simulink model "Training_Model_compactHEMS"  (R2023b)
settings: Solver=VariableStepAuto  StartTime=0.0  StopTime=runtime  RelTol=1e-3
undefined symbols (not defined in the file or in its folder): battery_capacity, battery_efficiency, battery_max_charge, battery_max_soc, battery_min_soc, battery_soc_initial, DiscIntNeverNeededParam, runtime, Ts
libraries: simulink x2, fuzblock x2, eeGeneralControl x1, dspstat3 x1, spspowerguiLib x1
settings Model: Creator=leons  LastModifiedBy=leons

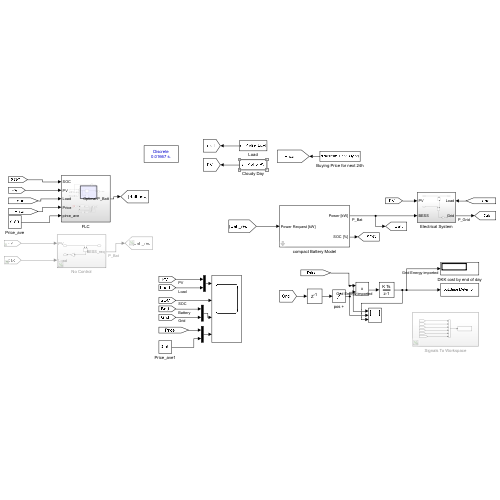
[thumbnail: Simulink's stored preview of the top-level diagram]
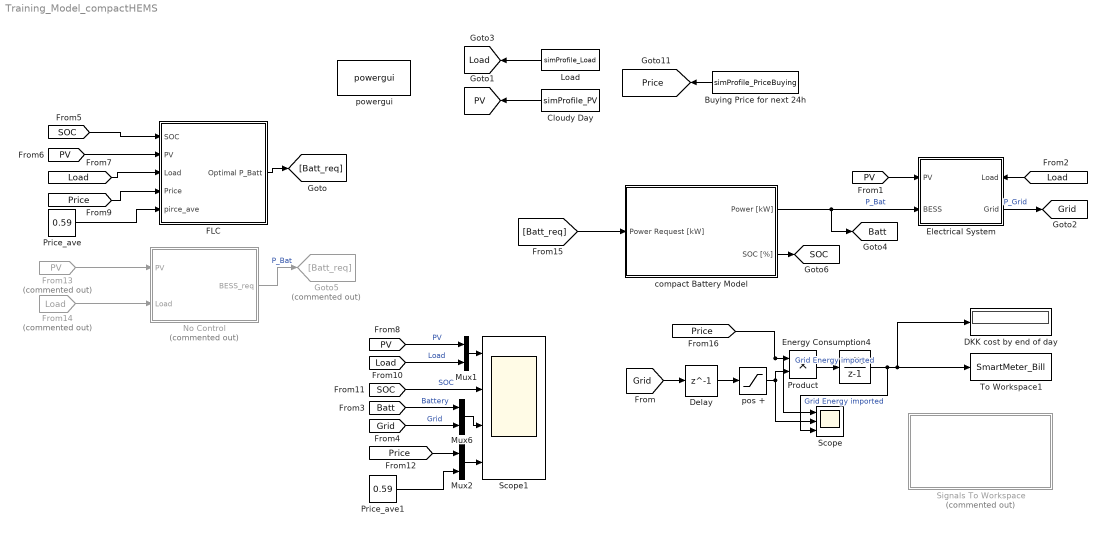
== system Training_Model_compactHEMS ==
  Buying Price for next 24h : FromWorkspace  VariableName=simProfile_PriceBuying  SampleTime=Ts*60  ZeroCross=off  OutputAfterFinalValue=Holding final value
  Cloudy Day : FromWorkspace  VariableName=simProfile_PV  ZeroCross=off
  DKK cost by end of day : Display
  Delay : Delay  DelayLength=1  SampleTime=Ts*60
  Electrical System : Subsystem
      settings: PortSchema="{\"entries\":[{\"content\":{\"sides\":[{\"content\":{\"connectorIds\":[\"In1\",\"Out1\"]},\"type\":\"ConnectorPlacement.EquallySpacedRectSide\",\"uuid\":\"ea2d6f6f-0b16-4ab1-9278-b701b85b7cf6\"},{\"content\":{\"connectorIds\":[\"In2\",\"In3\"],\"side\":\"RIGHT\"},\"type\":\"ConnectorPlacement.EquallySpacedRectSide\",\"uuid\":\"7f792676-012d-49e4-aa54-4a4cf568511b\"},{\"content\":{\"side\":\"TOP\"},\"type\":\"ConnectorPlacement.EquallySpacedRectSide\",\"uuid\":\"0f596cfa-1807-49b9-975a-a3b3036f9244\"}]},\"type\":\"ConnectorPlacement.EquallySpacedConnector\",\"uuid\":\"02bb58de-c0fd-4021-befc-2f3cc3c5a74e\"}],\"packageUris\":[\"http://schema.mathworks.com/mf0/Connector/R2020b\"],\"version\":\"1.0\"}"
  Energy Consumption4 : DiscreteIntegrator  gainval=1  SampleTime=Ts*60  ICPrevOutput=DiscIntNeverNeededParam  ICPrevScaledInput=DiscIntNeverNeededParam
  FLC : Subsystem
  From13 : From  Commented=on  GotoTag=PV  TagVisibility=global
  From14 : From  Commented=on  GotoTag=Load  TagVisibility=global
  Goto5 : Goto  Commented=on  GotoTag=Batt_req
  Load : FromWorkspace  VariableName=simProfile_Load  SampleTime=Ts  ZeroCross=off  OutputAfterFinalValue=Holding final value
  Mux1 : Mux  Inputs=2
  Mux2 : Mux  Inputs=2
  Mux6 : Mux  Inputs=2
  No Control : Subsystem  Commented=on
      settings: PortSchema="{\"entries\":[{\"content\":{\"sides\":[{\"content\":{\"connectorIds\":[\"Out1\"]},\"type\":\"ConnectorPlacement.EquallySpacedRectSide\",\"uuid\":\"ea2d6f6f-0b16-4ab1-9278-b701b85b7cf6\"},{\"content\":{\"connectorIds\":[\"In1\",\"In2\"],\"side\":\"RIGHT\"},\"type\":\"ConnectorPlacement.EquallySpacedRectSide\",\"uuid\":\"7f792676-012d-49e4-aa54-4a4cf568511b\"},{\"content\":{\"side\":\"TOP\"},\"type\":\"ConnectorPlacement.EquallySpacedRectSide\",\"uuid\":\"0f596cfa-1807-49b9-975a-a3b3036f9244\"}]},\"type\":\"ConnectorPlacement.EquallySpacedConnector\",\"uuid\":\"02bb58de-c0fd-4021-befc-2f3cc3c5a74e\"}],\"packageUris\":[\"http://schema.mathworks.com/mf0/Connector/R2020b\"],\"version\":\"1.0\"}"
  Price_ave : Constant  Value=0.59
  Price_ave1 : Constant  Value=0.59
  Product : Product
  Scope : Scope  NumInputPorts=3
  Scope1 : Scope  NumInputPorts=4
  Signals To Workspace : Subsystem  Commented=on
  To Workspace1 : ToWorkspace  VariableName=SmartMeter_Bill  SaveFormat=Structure With Time  SampleTime=-1
  compact Battery Model : Subsystem  mask{Pmax=battery_max_charge, Emax=battery_capacity, SOCinit=battery_soc_initial, Eff=battery_efficiency*100, SOCmax=battery_max_soc, SOCmin=battery_min_soc}
      mask prompts: Pmax "Max Power [kW] (both for charging and discharging)"; Emax "Total Storage Energy [kWh]"; SOCinit "Initial SOC [%]"; Eff "Round Trip Efficiency [%]"; SOCmax "SOC max"; SOCmin "SOC min"
  pos + : Saturate  UpperLimit=inf  LowerLimit=0  ZeroCross=off
  powergui : spspowerguiLib/powergui  Priority=1  SimulationMode=Discrete  SampleTime=Ts  frequency=60  Iterations=50  frequencyindice=60  Pbase=100e6  ErrMax=1e-4  UnitsV=kV  UnitsW=MW  buscounter=0  FunctionMessages=off  echomessages=off  EnableUseOfTLC=off  CurrentSourceSwitches=off  DisableSnubberDevices=off  DisableRonSwitches=off  DisableVfSwitches=off  DisplayEquations=off  AutomaticDiscreteSolvers=off  SolverType=Tustin/Backward Euler (TBE)  Interpol=off  ExternalGateDelay=off  methode=off  Ts=100  x0status=blocks  SPID=on  SwTol=0  HookPort=off  NonlinearTolerance=1e-4  nMaxIteration=100  ContinueOnMaxIteration=off  RestoreLinks=warning  ResistiveCurrentMeasurement=off  Frange=[0:2:500]  Ylog=off  Xlog=on  ShowGrid=off  save=off  variable=ZData  structure=0  ZoomFFT=off  StartTime=0.0  cycles=1  DisplayStyle=1  fundamental=60  FreqAxis=off  MaxFrequency=1000  frequencyindicesteady=1  RmsSteady=1  display=off
  tag scope: Batt=global, Grid=global, Load=global, PV=global, Price=global, SOC=global
  wires:
  [PV] -> FLC/2(PV)
  [Load] -> FLC/3(Load)
  [Price] -> FLC/4(Price)
  [SOC] -> FLC/1(SOC)
  Cloudy Day/1 -> [PV]
  Load/1 -> [Load]
  Buying Price for next 24h/1 -> [Price]
  compact Battery Model/2(SOC [%]) -> [SOC]
  compact Battery Model/1(Power [kW]) -> Electrical System/3(BESS), [Batt]  "P_Bat"
  [PV] -> Electrical System/2(PV)
  [Load] -> Electrical System/1(Load)
  Electrical System/1(Grid) -> [Grid]  "P_Grid"
  Product/1 -> Energy Consumption4/1  "Grid Energy imported"
  pos +/1 -> Scope/2, Product/2
  [Grid] -> Delay/1
  [Grid] -> Mux6/2  "Grid"
  [PV] -> Mux1/1  "PV"
  [Load] -> Mux1/2  "Load"
  Mux6/1 -> Scope1/3
  [Batt] -> Mux6/1  "Battery"
  [SOC] -> Scope1/2  "SOC"
  Mux1/1 -> Scope1/1
  [Price] -> Mux2/1
  From14/1 -> No Control/2(Load)
  From13/1 -> No Control/1(PV)
  FLC/1(Optimal P_Batt) -> [Batt_req]
  [Batt_req] -> compact Battery Model/1(Power Request [kW])
  No Control/1(BESS_req) -> Goto5/1  "P_Bat"
  Price_ave/1 -> FLC/5(pirce_ave)
  [Price] -> Scope/1, Product/1
  Delay/1 -> pos +/1
  Energy Consumption4/1 -> Scope/3, DKK cost by end of day/1, To Workspace1/1  "Grid Energy imported"
  Price_ave1/1 -> Mux2/2
  Mux2/1 -> Scope1/4

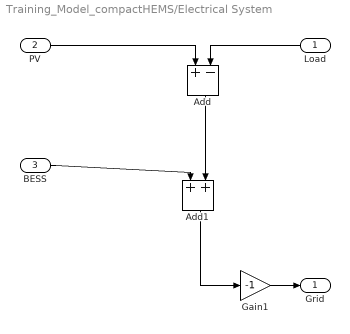
== system Training_Model_compactHEMS/Electrical System ==
  Load : Inport
  PV : Inport  Port=2
  BESS : Inport  Port=3
  Add : Sum  Inputs=+-
  Add1 : Sum
  Gain1 : Gain  Gain=-1
  Grid : Outport
  wires:
  Add/1 -> Add1/2
  BESS/1 -> Add1/1
  Load/1 -> Add/2
  Add1/1 -> Gain1/1
  PV/1 -> Add/1
  Gain1/1 -> Grid/1

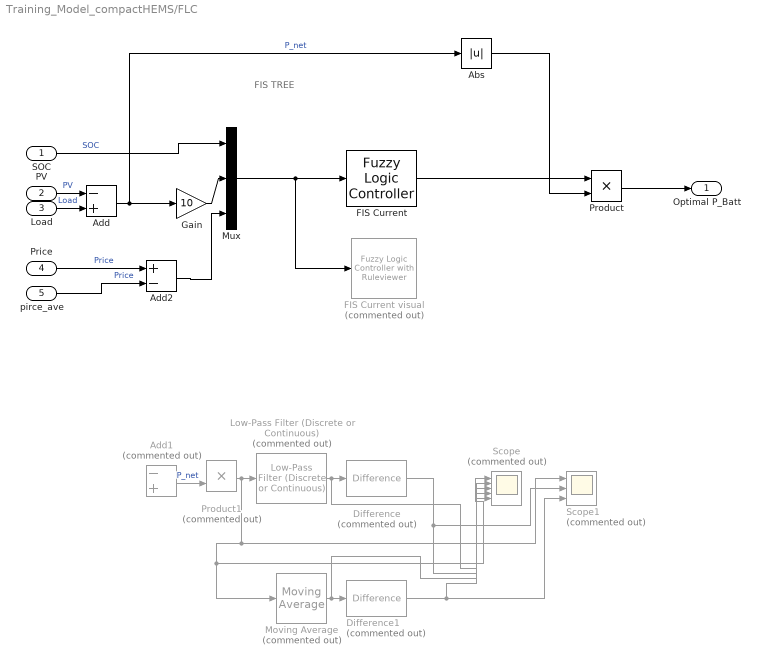
== system Training_Model_compactHEMS/FLC ==
  note: FIS TREE
  SOC : Inport
  PV : Inport  Port=2
  Load : Inport  Port=3
  Price : Inport  Port=4
  pirce_ave : Inport  Port=5
  Abs : Abs  SaturateOnIntegerOverflow=off
  Add : Sum  Inputs=-+
  Add1 : Sum  Commented=on  Inputs=-+
  Add2 : Sum  Inputs=+-
  Difference : simulink/Discrete/Difference  Commented=on  ICPrevInput=0.0  OutMin=[]  OutMax=[]  OutDataType=fixdt(1, 16)  OutScaling=2^-10  DoSatur=off
  Difference1 : simulink/Discrete/Difference  Commented=on  ICPrevInput=0.0  OutMin=[]  OutMax=[]  OutDataType=fixdt(1, 16)  OutScaling=2^-10  DoSatur=off
  FIS Current : fuzblock/Fuzzy Logic  Controller  FIS=fisT  OutputSampleNumber=runtime*1/Ts  DataType=double  FuzzifiedInputs=off  RuleFiringStrengths=off  RuleOutputs=off  AggregatedOutputs=off  SimulateUsing=Interpreted execution  OutOfRangeInputValueMessage=warning  NoRuleFiredMessage=warning  EmptyOutputFuzzySetMessage=warning
  FIS Current visual : fuzblock/Fuzzy Logic  Controller  with Ruleviewer  Commented=on  fismatrix=fis_Current  Ts=0.25
  Gain : Gain  Gain=10
  Low-Pass Filter (Discrete or Continuous) : eeGeneralControl/Low-Pass Filter (Discrete or Continuous)  Commented=on  K=1  T=1  B=inf  A=-inf  init_option=Inherited from block input  x0=0  Ts=0.25
  Moving Average : dspstat3/Moving Average  Commented=on  Method=Sliding window  ForgettingFactorPort=off  SpecifyWindowLength=on  WindowLength=5  OverlapLength=4  AllowArbitraryInputLength=off  ForgettingFactor=0.9  SimulateUsing=Code generation
  Mux : Mux  Inputs=3
  Product : Product
  Product1 : Product  Commented=on
  Scope : Scope  Commented=on  NumInputPorts=5
  Scope1 : Scope  Commented=on  NumInputPorts=3
  Optimal P_Batt : Outport  VectorParamsAs1DForOutWhenUnconnected=off
  wires:
  SOC/1 -> Mux/1  "SOC"
  PV/1 -> Add/1  "PV"
  Add/1 -> Abs/1, Gain/1  "P_net"
  Load/1 -> Add/2  "Load"
  Mux/1 -> FIS Current visual/1, FIS Current/1
  Price/1 -> Add2/1  "Price"
  Gain/1 -> Mux/2
  FIS Current/1 -> Product/1
  Product/1 -> Optimal P_Batt/1
  Abs/1 -> Product/2
  ? -> Add1/1  "PV_pred"
  ? -> Add1/2  "Load_pred"
  Add1/1 -> Product1/2  "P_net"
  Product1/1 -> Scope/1, Moving Average/1, Scope1/1, Low-Pass Filter (Discrete or Continuous)/1
  Low-Pass Filter (Discrete or Continuous)/1 -> Scope/2, Difference/1
  Difference/1 -> Scope1/2, Scope/3
  Moving Average/1 -> Scope/4, Difference1/1
  Difference1/1 -> Scope1/3, Scope/5
  pirce_ave/1 -> Add2/2  "Price"
  Add2/1 -> Mux/3

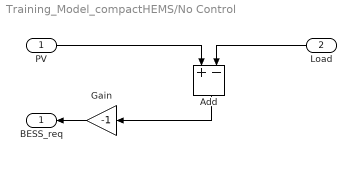
== system Training_Model_compactHEMS/No Control ==
  PV : Inport
  Load : Inport  Port=2
  Add : Sum  Inputs=+-
  Gain : Gain  Gain=-1
  BESS_req : Outport
  wires:
  Load/1 -> Add/2
  PV/1 -> Add/1
  Add/1 -> Gain/1
  Gain/1 -> BESS_req/1

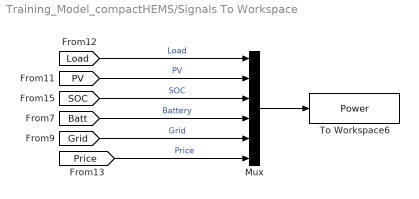
== system Training_Model_compactHEMS/Signals To Workspace ==
  Mux : Mux  Inputs=6
  To Workspace6 : ToWorkspace  VariableName=Power  SaveFormat=Structure With Time  SampleTime=-1
  wires:
  [PV] -> Mux/2  "PV"
  [SOC] -> Mux/3  "SOC"
  [Batt] -> Mux/4  "Battery"
  [Grid] -> Mux/5  "Grid"
  [Price] -> Mux/6  "Price"
  Mux/1 -> To Workspace6/1
  [Load] -> Mux/1  "Load"

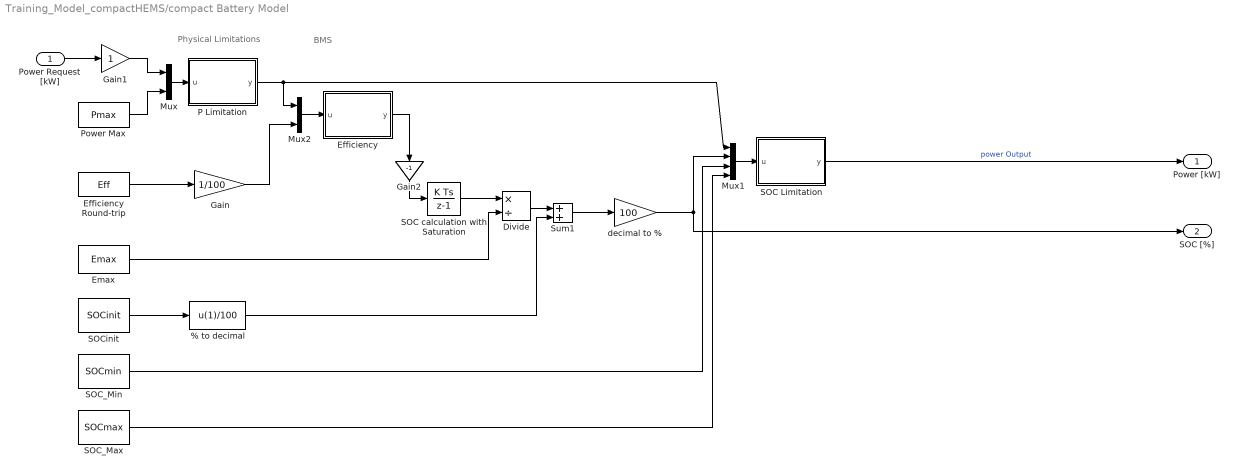
== system Training_Model_compactHEMS/compact Battery Model ==
  note: Physical Limitations
  note: BMS
  Power Request [kW] : Inport
  % to decimal : Fcn  Expr=u(1)/100
  Divide : Product  Inputs=*/
  Efficiency : MATLAB Function  TreatAsAtomicUnit=on
  Efficiency Round-trip : Constant  Value=Eff
  Emax : Constant  Value=Emax
  Gain : Gain  Gain=1/100
  Gain1 : Gain
  Gain2 : Gain  Gain=-1
  Mux : Mux  Inputs=2
  Mux1 : Mux
  Mux2 : Mux  Inputs=2
  P Limitation : MATLAB Function  TreatAsAtomicUnit=on
  Power Max : Constant  Value=Pmax
  SOC Limitation : MATLAB Function  TreatAsAtomicUnit=on
  SOC calculation with Saturation : DiscreteIntegrator  gainval=1  SampleTime=-1  LimitOutput=on  UpperSaturationLimit=SOCmax/100*Emax -SOCinit/100 *Emax  LowerSaturationLimit=+SOCmin/100*Emax - SOCinit/100 *Emax  ICPrevOutput=DiscIntNeverNeededParam  ICPrevScaledInput=DiscIntNeverNeededParam
  SOC_Max : Constant  Value=SOCmax
  SOC_Min : Constant  Value=SOCmin
  SOCinit : Constant  Value=SOCinit
  Sum1 : Sum
  decimal to % : Gain  Gain=100
  Power [kW] : Outport
  SOC [%] : Outport  Port=2
  wires:
  Mux/1 -> P Limitation/1(u)
  decimal to %/1 -> Mux1/2, SOC [%]/1
  Efficiency Round-trip/1 -> Gain/1
  SOCinit/1 -> % to decimal/1
  Sum1/1 -> decimal to %/1
  Divide/1 -> Sum1/1
  SOC calculation with Saturation/1 -> Divide/1
  % to decimal/1 -> Sum1/2
  Mux1/1 -> SOC Limitation/1(u)
  SOC Limitation/1(y) -> Power [kW]/1  "power Output"
  Gain2/1 -> SOC calculation with Saturation/1
  P Limitation/1(y) -> Mux2/1, Mux1/1
  Gain/1 -> Mux2/2
  Mux2/1 -> Efficiency/1(u)
  Emax/1 -> Divide/2
  SOC_Min/1 -> Mux1/3
  SOC_Max/1 -> Mux1/4
  Power Max/1 -> Mux/2
  Gain1/1 -> Mux/1
  Efficiency/1(y) -> Gain2/1
  Power Request [kW]/1 -> Gain1/1

== matlab function Training_Model_compactHEMS/compact Battery Model/SOC Limitation ==
  data: u input; y output
function y = fcn(u)
Pout = u(1);
SOC = u(2) ;
SOC_min = u(3);
SOC_max = u(4);

if ( SOC<=SOC_min || SOC>=SOC_max)
    Pout = 0;
end

y = Pout;

== matlab function Training_Model_compactHEMS/compact Battery Model/Efficiency ==
  data: u input; y output
function y = fcn(u)
Preq = u(1);
eff = u(2) ;

if ( Preq>0) % Discharging
    y = u(1)/u(2); % for charging soc = P_bat/eff
else % charging
    y = u(1)*u(2); % for charging soc = P_bat*eff
end

== matlab function Training_Model_compactHEMS/compact Battery Model/P Limitation ==
  data: u input; y output
function y = fcn(u)
y = min(max(u(1), -u(2)), u(2));
